simulink model "MARCH_v1_4"  (R2016a)
settings: Solver=FixedStepDiscrete  StartTime=0.0  StopTime=inf  FixedStep=0.001  RelTol=1e-3
PostLoadFcn:
  | build_location = fullfile(fileparts(which(bdroot)),'build');
  | 
  | set_param(0, 'CacheFolder', build_location);
  | set_param(0, 'CodeGenFolder', build_location);
InitFcn:
  | % Change dir to model location
  | cd(fileparts(which(bdroot)));
  | 
  | % Run init script
  | init_model;
  | 
  | load db.mat
  | initialize_model_param
StartFcn:
  | % Make sure we always move back to model folder
  | cd(fileparts(which(bdroot)));
StopFcn:
  | % Make sure we always move back to model folder
  | cd(fileparts(which(bdroot)));
model workspace (MAT data in the model file):
  localValue = 1
  targetValue = 0
libraries: xpcethercatlib x57, slrtlib x7, dspnetwork x1, aerolibanimutils x1
(part 2 of 2)

== matlab function MARCH_v1_4/Controllers/Transition Controller/Trajectory ==
  data: base input; q output; trigger input; q input size=[1 6]; debugOut output; debugIn input
function [q,debugOut]= fcn(base,trigger,q,debugIn)
%#codegen

persistent r splineCtrl i triggerPersistent trajectory fullStep hold;

%% Initialize all variables
if(isempty(splineCtrl))
    splineCtrl = splineController();
end


if(isempty(fullStep))
    fullStep = 0;
end

if(isempty(r))
    % Get frequency of the model
    r = robotics();
    r.base = base;
    
end

if(isempty(hold))
    hold = 0;
end

if(isempty(i))
    i = 0;
end

if(isempty(triggerPersistent))
    triggerPersistent = trigger;
end


if(isempty(trajectory))
    trajectory = [0 0];
end

%% Logic
% Only run this for the beginning of the swing
r.torso_z = debugIn;

% Reset values if trigger is toggled.
if(triggerPersistent ~= trigger)
    r.resetTorso();
    r.switchFoot(r.base);
    i = 0;
    hold = 0;
    triggerPersistent = trigger;
end

if(trigger == -1)
   fullStep = 0; 
end

% Hold exoskeleton in same position after a single step
if(hold)
    debugOut = r.torso_z;
    q = r.q;
    return
end

if(~i)
    
    % We set the method of whether we want an analytically generated spline
    % or a spline directly from the database.
    % Options: 'analytical' and 'database'
    if(~fullStep)
        trajectory = splineCtrl.method('analytical').getHalfStep();
        fullStep = 1;
    else
        trajectory = splineCtrl.method('analytical').getFullStep();
    end
    
    % Transform the spline to the correct frame based on which foot is
    % swinging
    trajectory = r.transformSpline(trajectory);
    
    i = i+1;
end

r.point = [trajectory(1,i) trajectory(2,i) trajectory(3,i)];

r.stepPosture();
r.inverseKinematics();

q = r.q;
debugOut = r.torso_z;

% Set final values as initial values for the next iteration
r.refresh();

% Reset iterator after we're done with the trajectory, otherwise we
% increment the counter and continue iterating as simulink continues
% sampling
if( i < (length(trajectory)))
    i = i+1;
else
    hold = 1;
end

end

== matlab function MARCH_v1_4/Controllers/Point & Go/Torso Trajectory ==
  data: desired input; current input; z output
function z = fcn(desired, current)
%#codegen

persistent trajectory i desiredPersistent;

% Speed at which we home in SAMPLES
samples = 1000;

if (isempty(i))
    i = 0;
    
    % Hack to fix initial condition of delay during init phase
    current = desired;
end

if(isempty(desiredPersistent))
    desiredPersistent = desired;
end

if(isempty(trajectory))
    trajectory = linspace(current,desiredPersistent,samples);
end

if(desiredPersistent ~= desired)
    trajectory = linspace(current,desired,samples);
    desiredPersistent = desired;
    i = 0;
end

if(i < samples)
    i = i+1;
end

z = trajectory(i);

== matlab function MARCH_v1_4/Controllers/Point & Go/Trajectory ==
  data: base input; q output; trigger input; point input; q input size=[1 6]; debugOut output; debugIn input
function [q,debugOut]= fcn(base,trigger, point,q,debugIn)
%#codegen

persistent r splineCtrl i triggerPersistent trajectory fullStep hold pointPersistent;

%% Initialize all variables
if(isempty(splineCtrl))
    splineCtrl = splineController();
end


if(isempty(fullStep))
    fullStep = 0;
end

if(isempty(r))
    r = robotics();
    r.base = base;
    
end

if(isempty(hold))
    hold = 0;
end

if(isempty(i))
    i = 0;
end

if(isempty(triggerPersistent))
    triggerPersistent = trigger;
end

if(isempty(pointPersistent))
    pointPersistent = point;
end

if(isempty(trajectory))
    trajectory = [0 0];
end

%% Logic
% Only run this for the beginning of the swing
r.torso_z = debugIn;

% Reset values if trigger is toggled.
if(triggerPersistent ~= trigger)
    r.resetTorso();
    r.base = base;
    i = 0;
    hold = 0;
    triggerPersistent = trigger;
end


% Hold exoskeleton in same position after a single step
if(hold)
    debugOut = r.torso_z;
    q = r.q;
    return
end

if(~i)
    
    % We set the method of whether we want an analytically generated spline
    % or a spline directly from the database.
    % Options: 'analytical' and 'database'
    trajectory = splineCtrl.method('analytical').getStepFromPoint(point);
    
    
    
    % Transform the spline to the correct frame based on which foot is
    % swinging
    trajectory = r.transformSpline(trajectory);
    
    i = i+1;
end

r.point = [trajectory(1,i) trajectory(2,i) trajectory(3,i)];

r.stepPosture();
r.inverseKinematics();

q = r.q;
debugOut = r.torso_z;

% Set final values as initial values for the next iteration
r.refresh();

% Reset iterator after we're done with the trajectory, otherwise we
% increment the counter and continue iterating as simulink continues
% sampling
if( i < (length(trajectory)))
    i = i+1;
else
    hold = 1;
end

end

== matlab function MARCH_v1_4/Controllers/Sit and Stand/Torso Trajectory ==
  data: desired input; current input; z output
function z = fcn(desired, current)
%#codegen

persistent trajectory i desiredPersistent;

% Speed at which we home in SAMPLES
samples = 1000;

if (isempty(i))
    i = 0;
    
    % Hack to fix initial condition of delay during init phase
    current = desired;
end

if(isempty(desiredPersistent))
    desiredPersistent = desired;
end

if(isempty(trajectory))
    trajectory = linspace(current,desiredPersistent,samples);
end

if(desiredPersistent ~= desired)
    trajectory = linspace(current,desired,samples);
    desiredPersistent = desired;
    i = 0;
end

if(i < samples)
    i = i+1;
end

z = trajectory(i);

== matlab function MARCH_v1_4/EtherCAT Joint Setpoints/exoskeleton/MATLAB Function ==
  data: jointAngle input; encVal output; par parameter
function encVal = convertToEncoderValues(jointAngle, par)
encVal = zeros(6,1);

for i = 1:6
    encVal(i) = rad2enc(jointAngle(i), i, par);
end

== matlab function MARCH_v1_4/Controllers/Sit and Stand/Trajectory ==
  data: stance input; q output; trigger input; q input size=[1 6]; debugOut output; debugIn input
function [q,debugOut]= fcn(stance,trigger,q,debugIn)
%#codegen

persistent r splineCtrl i triggerPersistent trajectory fullStep hold;

%% Initialize all variables
if(isempty(splineCtrl))
    splineCtrl = splineController();
end


if(isempty(fullStep))
    fullStep = 0;
end

if(isempty(r))
    % Get frequency of the model
    r = robotics();
    
end

if(isempty(hold))
    hold = 0;
end

if(isempty(i))
    i = 0;
end

if(isempty(triggerPersistent))
    triggerPersistent = trigger;
end


if(isempty(trajectory))
    trajectory = [0 0];
end

%% Logic
% Only run this for the beginning of the swing
r.torso_z = debugIn;
r.base = 1;

% Reset values if trigger is toggled.
if(triggerPersistent ~= trigger)
    r.resetTorso();
    i = 0;
    hold = 0;
    triggerPersistent = trigger;
end

if(trigger == -1)
    fullStep = 0;
end

% Hold exoskeleton in same position after a single step
if(hold)
    debugOut = r.torso_z;
    q = r.q;
    return
end

if(~i)
    
    % We set the method of whether we want an analytically generated spline
    % or a spline directly from the database.
    % Options: 'analytical' and 'database'
    if(~fullStep)
        trajectory = splineCtrl.method('analytical').getHalfStep();
        fullStep = 1;
    else
        trajectory = splineCtrl.method('analytical').getFullStep();
    end
    
    % Transform the spline to the correct frame based on which foot is
    % swinging
    trajectory = r.transformSpline(trajectory);
    
    i = i+1;
end

r.point = [trajectory(1,1) trajectory(2,1) trajectory(3,1)];
r.stepPosture();
r.inverseKinematics();

q = r.q;
debugOut = r.torso_z;

% Set final values as initial values for the next iteration
r.refresh();

% Reset iterator after we're done with the trajectory, otherwise we
% increment the counter and continue iterating as simulink continues
% sampling
if( i < 10000)
    i = i+1;
else
    i = 0;
%     hold = 1;
end

end
